simulink model "TST_DrvDem_SetPoint"  (R2016b)
settings: Solver=FixedStepDiscrete  StartTime=0.0  StopTime=simTime  FixedStep=sampleTime  RelTol=1e-3
values from neighbouring files (symbols this model uses):
  testCase = 1    [initTST_DrvDem_SetPoint_001.m]    (also in initTST_DrvDem_SetPoint_002.m = 2; initTST_DrvDem_SetPoint_003.m = 3)
libraries: simulink x13, UnitTest_Lib x9
settings Model: Creator=zhengjinyan  LastModifiedBy=zhengjinyan
settings DebuggingCC: SignalRangeChecking=error

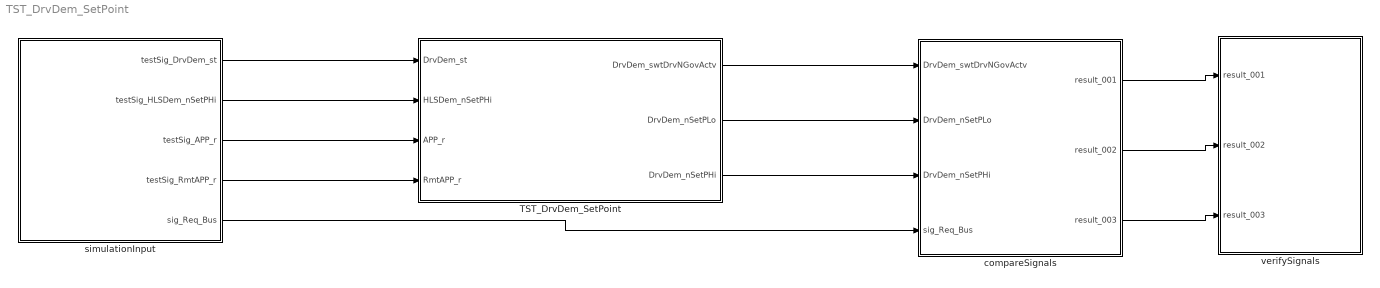
== system TST_DrvDem_SetPoint ==
  TST_DrvDem_SetPoint : Subsystem
  compareSignals : Subsystem
  simulationInput : Subsystem
  verifySignals : Subsystem
  wires:
  simulationInput/1(testSig_DrvDem_st) -> TST_DrvDem_SetPoint/1(DrvDem_st)
  simulationInput/2(testSig_HLSDem_nSetPHi) -> TST_DrvDem_SetPoint/2(HLSDem_nSetPHi)
  simulationInput/3(testSig_APP_r) -> TST_DrvDem_SetPoint/3(APP_r)
  simulationInput/4(testSig_RmtAPP_r) -> TST_DrvDem_SetPoint/4(RmtAPP_r)
  TST_DrvDem_SetPoint/1(DrvDem_swtDrvNGovActv) -> compareSignals/1(DrvDem_swtDrvNGovActv)
  TST_DrvDem_SetPoint/2(DrvDem_nSetPLo) -> compareSignals/2(DrvDem_nSetPLo)
  TST_DrvDem_SetPoint/3(DrvDem_nSetPHi) -> compareSignals/3(DrvDem_nSetPHi)
  simulationInput/5(sig_Req_Bus) -> compareSignals/4(sig_Req_Bus)
  compareSignals/1(result_001) -> verifySignals/1(result_001)
  compareSignals/2(result_002) -> verifySignals/2(result_002)
  compareSignals/3(result_003) -> verifySignals/3(result_003)

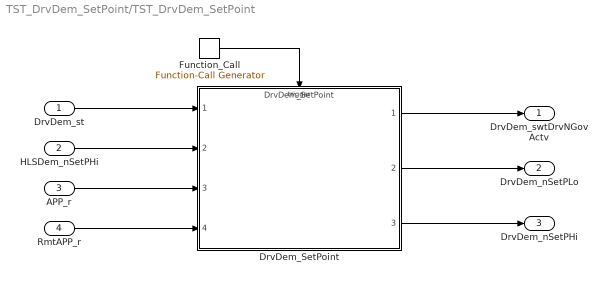
== system TST_DrvDem_SetPoint/TST_DrvDem_SetPoint ==
  DrvDem_st : Inport
  HLSDem_nSetPHi : Inport  Port=2
  APP_r : Inport  Port=3
  RmtAPP_r : Inport  Port=4
  DrvDem_SetPoint : ModelReference  ModelNameDialog=DrvDem_SetPoint  SimulationMode=Normal  ModelReferenceVersion=1.79  TriggerPortName=function  TriggerPortTriggerType=function-call  TriggerPortStatesWhenEnabling=held
  Function_Call : simulink/Ports & Subsystems/Function-Call Generator  sample_time=sampleTime  numberOfIterations=1
  DrvDem_swtDrvNGovActv : Outport
  DrvDem_nSetPLo : Outport  Port=2
  DrvDem_nSetPHi : Outport  Port=3
  wires:
  Function_Call/1 -> DrvDem_SetPoint/Trigger
  DrvDem_st/1 -> DrvDem_SetPoint/1
  HLSDem_nSetPHi/1 -> DrvDem_SetPoint/2
  APP_r/1 -> DrvDem_SetPoint/3
  RmtAPP_r/1 -> DrvDem_SetPoint/4
  DrvDem_SetPoint/1 -> DrvDem_swtDrvNGovActv/1
  DrvDem_SetPoint/2 -> DrvDem_nSetPLo/1
  DrvDem_SetPoint/3 -> DrvDem_nSetPHi/1

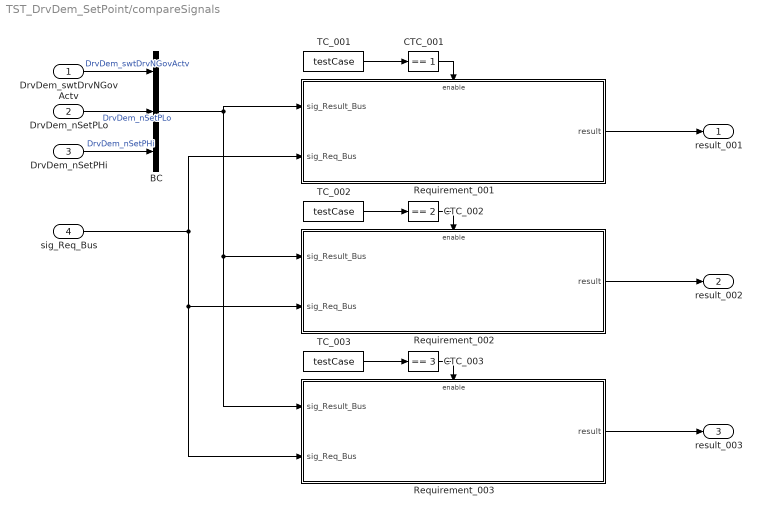
== system TST_DrvDem_SetPoint/compareSignals ==
  DrvDem_swtDrvNGovActv : Inport
  DrvDem_nSetPLo : Inport  Port=2
  DrvDem_nSetPHi : Inport  Port=3
  sig_Req_Bus : Inport  Port=4
  BC : BusCreator  Inputs=3
  CTC_001 : simulink/Logic and Bit Operations/Compare To Constant  relop===  const=1  OutDataTypeStr=boolean
  CTC_002 : simulink/Logic and Bit Operations/Compare To Constant  relop===  const=2  OutDataTypeStr=boolean
  CTC_003 : simulink/Logic and Bit Operations/Compare To Constant  relop===  const=3  OutDataTypeStr=boolean
  Requirement_001 : Subsystem
  Requirement_002 : Subsystem
  Requirement_003 : Subsystem
  TC_001 : Constant  Value=testCase
  TC_002 : Constant  Value=testCase
  TC_003 : Constant  Value=testCase
  result_001 : Outport
  result_002 : Outport  Port=2
  result_003 : Outport  Port=3
  wires:
  DrvDem_swtDrvNGovActv/1 -> BC/1  "DrvDem_swtDrvNGovActv"
  DrvDem_nSetPLo/1 -> BC/2  "DrvDem_nSetPLo"
  DrvDem_nSetPHi/1 -> BC/3  "DrvDem_nSetPHi"
  TC_001/1 -> CTC_001/1
  CTC_001/1 -> Requirement_001/Enable
  sig_Req_Bus/1 -> Requirement_002/2(sig_Req_Bus), Requirement_003/2(sig_Req_Bus), Requirement_001/2(sig_Req_Bus)
  BC/1 -> Requirement_002/1(sig_Result_Bus), Requirement_003/1(sig_Result_Bus), Requirement_001/1(sig_Result_Bus)
  Requirement_001/1(result) -> result_001/1
  TC_002/1 -> CTC_002/1
  CTC_002/1 -> Requirement_002/Enable
  Requirement_002/1(result) -> result_002/1
  TC_003/1 -> CTC_003/1
  CTC_003/1 -> Requirement_003/Enable
  Requirement_003/1(result) -> result_003/1

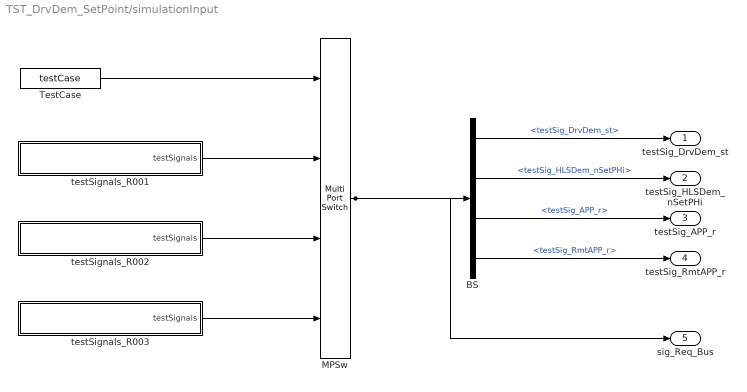
== system TST_DrvDem_SetPoint/simulationInput ==
  BS : BusSelector  OutputSignals=testSig_DrvDem_st,testSig_HLSDem_nSetPHi,testSig_APP_r,testSig_RmtAPP_r
  MPSw : MultiPortSwitch  SaturateOnIntegerOverflow=on  InputSameDT=on
  TestCase : Constant  Value=testCase
  testSignals_R001 : Subsystem
  testSignals_R002 : Subsystem
  testSignals_R003 : Subsystem
  testSig_DrvDem_st : Outport
  testSig_HLSDem_nSetPHi : Outport  Port=2
  testSig_APP_r : Outport  Port=3
  testSig_RmtAPP_r : Outport  Port=4
  sig_Req_Bus : Outport  Port=5
  wires:
  BS/1 -> testSig_DrvDem_st/1  "<testSig_DrvDem_st>"
  BS/2 -> testSig_HLSDem_nSetPHi/1  "<testSig_HLSDem_nSetPHi>"
  BS/3 -> testSig_APP_r/1  "<testSig_APP_r>"
  BS/4 -> testSig_RmtAPP_r/1  "<testSig_RmtAPP_r>"
  MPSw/1 -> BS/1, sig_Req_Bus/1
  TestCase/1 -> MPSw/1
  testSignals_R001/1(testSignals) -> MPSw/2
  testSignals_R002/1(testSignals) -> MPSw/3
  testSignals_R003/1(testSignals) -> MPSw/4

== system TST_DrvDem_SetPoint/verifySignals ==
  result_001 : Inport
  result_002 : Inport  Port=2
  result_003 : Inport  Port=3
  Assertion_001 : Assertion  Enabled=off
  Assertion_002 : Assertion  Enabled=off
  Assertion_003 : Assertion  Enabled=off
  wires:
  result_001/1 -> Assertion_001/1
  result_002/1 -> Assertion_002/1
  result_003/1 -> Assertion_003/1

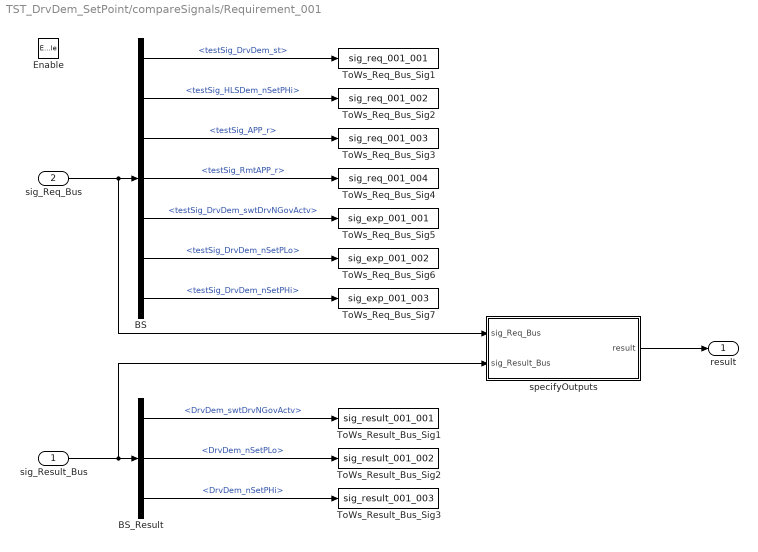
== system TST_DrvDem_SetPoint/compareSignals/Requirement_001 ==
  sig_Result_Bus : Inport
  sig_Req_Bus : Inport  Port=2
  Enable : EnablePort
  BS : BusSelector  OutputSignals=testSig_DrvDem_st,testSig_HLSDem_nSetPHi,testSig_APP_r,testSig_RmtAPP_r,testSig_DrvDem_swtDrvNGovActv,testSig_DrvDem_nSetPLo,testSig_DrvDem_nSetPHi
  BS_Result : BusSelector  OutputSignals=DrvDem_swtDrvNGovActv,DrvDem_nSetPLo,DrvDem_nSetPHi
  ToWs_Req_Bus_Sig1 : ToWorkspace  VariableName=sig_req_001_001  SaveFormat=Structure With Time
  ToWs_Req_Bus_Sig2 : ToWorkspace  VariableName=sig_req_001_002  SaveFormat=Structure With Time
  ToWs_Req_Bus_Sig3 : ToWorkspace  VariableName=sig_req_001_003  SaveFormat=Structure With Time
  ToWs_Req_Bus_Sig4 : ToWorkspace  VariableName=sig_req_001_004  SaveFormat=Structure With Time
  ToWs_Req_Bus_Sig5 : ToWorkspace  VariableName=sig_exp_001_001  SaveFormat=Structure With Time
  ToWs_Req_Bus_Sig6 : ToWorkspace  VariableName=sig_exp_001_002  SaveFormat=Structure With Time
  ToWs_Req_Bus_Sig7 : ToWorkspace  VariableName=sig_exp_001_003  SaveFormat=Structure With Time
  ToWs_Result_Bus_Sig1 : ToWorkspace  VariableName=sig_result_001_001  SaveFormat=Structure With Time
  ToWs_Result_Bus_Sig2 : ToWorkspace  VariableName=sig_result_001_002  SaveFormat=Structure With Time
  ToWs_Result_Bus_Sig3 : ToWorkspace  VariableName=sig_result_001_003  SaveFormat=Structure With Time
  specifyOutputs : Subsystem
  result : Outport
  wires:
  sig_Req_Bus/1 -> BS/1, specifyOutputs/1(sig_Req_Bus)
  BS/1 -> ToWs_Req_Bus_Sig1/1  "<testSig_DrvDem_st>"
  BS/2 -> ToWs_Req_Bus_Sig2/1  "<testSig_HLSDem_nSetPHi>"
  BS/3 -> ToWs_Req_Bus_Sig3/1  "<testSig_APP_r>"
  BS/4 -> ToWs_Req_Bus_Sig4/1  "<testSig_RmtAPP_r>"
  BS/5 -> ToWs_Req_Bus_Sig5/1  "<testSig_DrvDem_swtDrvNGovActv>"
  BS/6 -> ToWs_Req_Bus_Sig6/1  "<testSig_DrvDem_nSetPLo>"
  BS/7 -> ToWs_Req_Bus_Sig7/1  "<testSig_DrvDem_nSetPHi>"
  sig_Result_Bus/1 -> BS_Result/1, specifyOutputs/2(sig_Result_Bus)
  BS_Result/1 -> ToWs_Result_Bus_Sig1/1  "<DrvDem_swtDrvNGovActv>"
  BS_Result/2 -> ToWs_Result_Bus_Sig2/1  "<DrvDem_nSetPLo>"
  BS_Result/3 -> ToWs_Result_Bus_Sig3/1  "<DrvDem_nSetPHi>"
  specifyOutputs/1(result) -> result/1

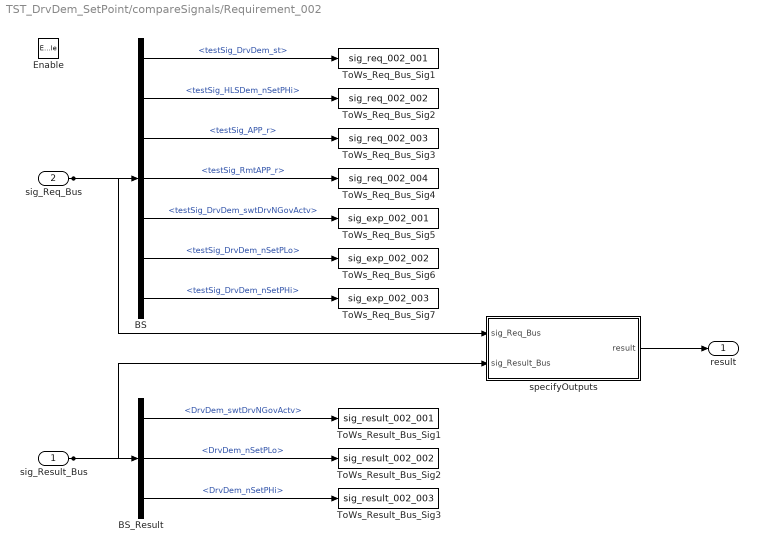
== system TST_DrvDem_SetPoint/compareSignals/Requirement_002 ==
  sig_Result_Bus : Inport
  sig_Req_Bus : Inport  Port=2
  Enable : EnablePort
  BS : BusSelector  OutputSignals=testSig_DrvDem_st,testSig_HLSDem_nSetPHi,testSig_APP_r,testSig_RmtAPP_r,testSig_DrvDem_swtDrvNGovActv,testSig_DrvDem_nSetPLo,testSig_DrvDem_nSetPHi
  BS_Result : BusSelector  OutputSignals=DrvDem_swtDrvNGovActv,DrvDem_nSetPLo,DrvDem_nSetPHi
  ToWs_Req_Bus_Sig1 : ToWorkspace  VariableName=sig_req_002_001  SaveFormat=Structure With Time
  ToWs_Req_Bus_Sig2 : ToWorkspace  VariableName=sig_req_002_002  SaveFormat=Structure With Time
  ToWs_Req_Bus_Sig3 : ToWorkspace  VariableName=sig_req_002_003  SaveFormat=Structure With Time
  ToWs_Req_Bus_Sig4 : ToWorkspace  VariableName=sig_req_002_004  SaveFormat=Structure With Time
  ToWs_Req_Bus_Sig5 : ToWorkspace  VariableName=sig_exp_002_001  SaveFormat=Structure With Time
  ToWs_Req_Bus_Sig6 : ToWorkspace  VariableName=sig_exp_002_002  SaveFormat=Structure With Time
  ToWs_Req_Bus_Sig7 : ToWorkspace  VariableName=sig_exp_002_003  SaveFormat=Structure With Time
  ToWs_Result_Bus_Sig1 : ToWorkspace  VariableName=sig_result_002_001  SaveFormat=Structure With Time
  ToWs_Result_Bus_Sig2 : ToWorkspace  VariableName=sig_result_002_002  SaveFormat=Structure With Time
  ToWs_Result_Bus_Sig3 : ToWorkspace  VariableName=sig_result_002_003  SaveFormat=Structure With Time
  specifyOutputs : Subsystem
  result : Outport
  wires:
  sig_Req_Bus/1 -> BS/1, specifyOutputs/1(sig_Req_Bus)
  BS/1 -> ToWs_Req_Bus_Sig1/1  "<testSig_DrvDem_st>"
  BS/2 -> ToWs_Req_Bus_Sig2/1  "<testSig_HLSDem_nSetPHi>"
  BS/3 -> ToWs_Req_Bus_Sig3/1  "<testSig_APP_r>"
  BS/4 -> ToWs_Req_Bus_Sig4/1  "<testSig_RmtAPP_r>"
  BS/5 -> ToWs_Req_Bus_Sig5/1  "<testSig_DrvDem_swtDrvNGovActv>"
  BS/6 -> ToWs_Req_Bus_Sig6/1  "<testSig_DrvDem_nSetPLo>"
  BS/7 -> ToWs_Req_Bus_Sig7/1  "<testSig_DrvDem_nSetPHi>"
  sig_Result_Bus/1 -> BS_Result/1, specifyOutputs/2(sig_Result_Bus)
  BS_Result/1 -> ToWs_Result_Bus_Sig1/1  "<DrvDem_swtDrvNGovActv>"
  BS_Result/2 -> ToWs_Result_Bus_Sig2/1  "<DrvDem_nSetPLo>"
  BS_Result/3 -> ToWs_Result_Bus_Sig3/1  "<DrvDem_nSetPHi>"
  specifyOutputs/1(result) -> result/1

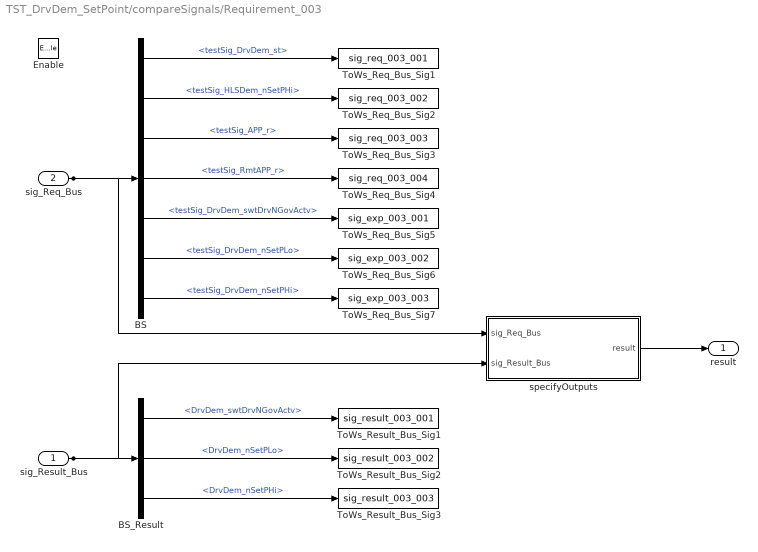
== system TST_DrvDem_SetPoint/compareSignals/Requirement_003 ==
  sig_Result_Bus : Inport
  sig_Req_Bus : Inport  Port=2
  Enable : EnablePort
  BS : BusSelector  OutputSignals=testSig_DrvDem_st,testSig_HLSDem_nSetPHi,testSig_APP_r,testSig_RmtAPP_r,testSig_DrvDem_swtDrvNGovActv,testSig_DrvDem_nSetPLo,testSig_DrvDem_nSetPHi
  BS_Result : BusSelector  OutputSignals=DrvDem_swtDrvNGovActv,DrvDem_nSetPLo,DrvDem_nSetPHi
  ToWs_Req_Bus_Sig1 : ToWorkspace  VariableName=sig_req_003_001  SaveFormat=Structure With Time
  ToWs_Req_Bus_Sig2 : ToWorkspace  VariableName=sig_req_003_002  SaveFormat=Structure With Time
  ToWs_Req_Bus_Sig3 : ToWorkspace  VariableName=sig_req_003_003  SaveFormat=Structure With Time
  ToWs_Req_Bus_Sig4 : ToWorkspace  VariableName=sig_req_003_004  SaveFormat=Structure With Time
  ToWs_Req_Bus_Sig5 : ToWorkspace  VariableName=sig_exp_003_001  SaveFormat=Structure With Time
  ToWs_Req_Bus_Sig6 : ToWorkspace  VariableName=sig_exp_003_002  SaveFormat=Structure With Time
  ToWs_Req_Bus_Sig7 : ToWorkspace  VariableName=sig_exp_003_003  SaveFormat=Structure With Time
  ToWs_Result_Bus_Sig1 : ToWorkspace  VariableName=sig_result_003_001  SaveFormat=Structure With Time
  ToWs_Result_Bus_Sig2 : ToWorkspace  VariableName=sig_result_003_002  SaveFormat=Structure With Time
  ToWs_Result_Bus_Sig3 : ToWorkspace  VariableName=sig_result_003_003  SaveFormat=Structure With Time
  specifyOutputs : Subsystem
  result : Outport
  wires:
  sig_Req_Bus/1 -> BS/1, specifyOutputs/1(sig_Req_Bus)
  BS/1 -> ToWs_Req_Bus_Sig1/1  "<testSig_DrvDem_st>"
  BS/2 -> ToWs_Req_Bus_Sig2/1  "<testSig_HLSDem_nSetPHi>"
  BS/3 -> ToWs_Req_Bus_Sig3/1  "<testSig_APP_r>"
  BS/4 -> ToWs_Req_Bus_Sig4/1  "<testSig_RmtAPP_r>"
  BS/5 -> ToWs_Req_Bus_Sig5/1  "<testSig_DrvDem_swtDrvNGovActv>"
  BS/6 -> ToWs_Req_Bus_Sig6/1  "<testSig_DrvDem_nSetPLo>"
  BS/7 -> ToWs_Req_Bus_Sig7/1  "<testSig_DrvDem_nSetPHi>"
  sig_Result_Bus/1 -> BS_Result/1, specifyOutputs/2(sig_Result_Bus)
  BS_Result/1 -> ToWs_Result_Bus_Sig1/1  "<DrvDem_swtDrvNGovActv>"
  BS_Result/2 -> ToWs_Result_Bus_Sig2/1  "<DrvDem_nSetPLo>"
  BS_Result/3 -> ToWs_Result_Bus_Sig3/1  "<DrvDem_nSetPHi>"
  specifyOutputs/1(result) -> result/1

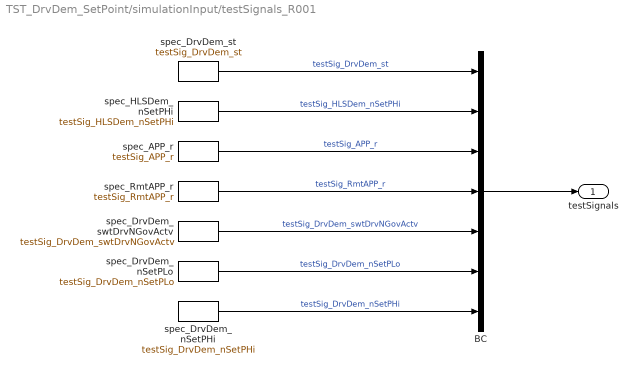
== system TST_DrvDem_SetPoint/simulationInput/testSignals_R001 ==
  BC : BusCreator  Inputs=7
  spec_APP_r : FromWorkspace  VariableName=testSig_APP_r  Interpolate=off  OutputAfterFinalValue=Holding final value
  spec_DrvDem_nSetPHi : FromWorkspace  VariableName=testSig_DrvDem_nSetPHi  Interpolate=off  OutputAfterFinalValue=Holding final value
  spec_DrvDem_nSetPLo : FromWorkspace  VariableName=testSig_DrvDem_nSetPLo  Interpolate=off  OutputAfterFinalValue=Holding final value
  spec_DrvDem_st : FromWorkspace  VariableName=testSig_DrvDem_st  Interpolate=off  OutputAfterFinalValue=Holding final value
  spec_DrvDem_swtDrvNGovActv : FromWorkspace  VariableName=testSig_DrvDem_swtDrvNGovActv  Interpolate=off  OutputAfterFinalValue=Holding final value
  spec_HLSDem_nSetPHi : FromWorkspace  VariableName=testSig_HLSDem_nSetPHi  Interpolate=off  OutputAfterFinalValue=Holding final value
  spec_RmtAPP_r : FromWorkspace  VariableName=testSig_RmtAPP_r  Interpolate=off  OutputAfterFinalValue=Holding final value
  testSignals : Outport
  wires:
  BC/1 -> testSignals/1
  spec_DrvDem_st/1 -> BC/1  "testSig_DrvDem_st"
  spec_HLSDem_nSetPHi/1 -> BC/2  "testSig_HLSDem_nSetPHi"
  spec_APP_r/1 -> BC/3  "testSig_APP_r"
  spec_RmtAPP_r/1 -> BC/4  "testSig_RmtAPP_r"
  spec_DrvDem_swtDrvNGovActv/1 -> BC/5  "testSig_DrvDem_swtDrvNGovActv"
  spec_DrvDem_nSetPLo/1 -> BC/6  "testSig_DrvDem_nSetPLo"
  spec_DrvDem_nSetPHi/1 -> BC/7  "testSig_DrvDem_nSetPHi"

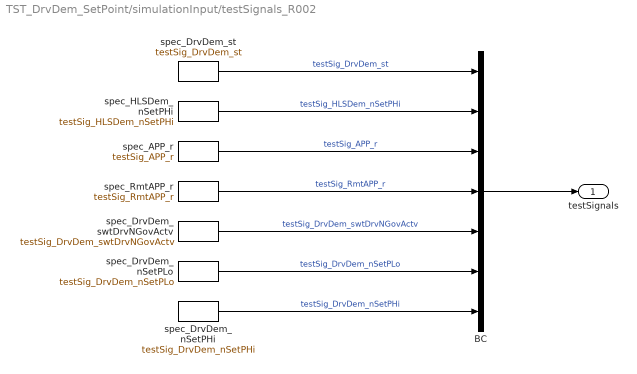
== system TST_DrvDem_SetPoint/simulationInput/testSignals_R002 ==
  BC : BusCreator  Inputs=7
  spec_APP_r : FromWorkspace  VariableName=testSig_APP_r  Interpolate=off  OutputAfterFinalValue=Holding final value
  spec_DrvDem_nSetPHi : FromWorkspace  VariableName=testSig_DrvDem_nSetPHi  Interpolate=off  OutputAfterFinalValue=Holding final value
  spec_DrvDem_nSetPLo : FromWorkspace  VariableName=testSig_DrvDem_nSetPLo  Interpolate=off  OutputAfterFinalValue=Holding final value
  spec_DrvDem_st : FromWorkspace  VariableName=testSig_DrvDem_st  Interpolate=off  OutputAfterFinalValue=Holding final value
  spec_DrvDem_swtDrvNGovActv : FromWorkspace  VariableName=testSig_DrvDem_swtDrvNGovActv  Interpolate=off  OutputAfterFinalValue=Holding final value
  spec_HLSDem_nSetPHi : FromWorkspace  VariableName=testSig_HLSDem_nSetPHi  Interpolate=off  OutputAfterFinalValue=Holding final value
  spec_RmtAPP_r : FromWorkspace  VariableName=testSig_RmtAPP_r  Interpolate=off  OutputAfterFinalValue=Holding final value
  testSignals : Outport
  wires:
  BC/1 -> testSignals/1
  spec_DrvDem_st/1 -> BC/1  "testSig_DrvDem_st"
  spec_HLSDem_nSetPHi/1 -> BC/2  "testSig_HLSDem_nSetPHi"
  spec_APP_r/1 -> BC/3  "testSig_APP_r"
  spec_RmtAPP_r/1 -> BC/4  "testSig_RmtAPP_r"
  spec_DrvDem_swtDrvNGovActv/1 -> BC/5  "testSig_DrvDem_swtDrvNGovActv"
  spec_DrvDem_nSetPLo/1 -> BC/6  "testSig_DrvDem_nSetPLo"
  spec_DrvDem_nSetPHi/1 -> BC/7  "testSig_DrvDem_nSetPHi"

== system TST_DrvDem_SetPoint/simulationInput/testSignals_R003 ==
  BC : BusCreator  Inputs=7
  spec_APP_r : FromWorkspace  VariableName=testSig_APP_r  Interpolate=off  OutputAfterFinalValue=Holding final value
  spec_DrvDem_nSetPHi : FromWorkspace  VariableName=testSig_DrvDem_nSetPHi  Interpolate=off  OutputAfterFinalValue=Holding final value
  spec_DrvDem_nSetPLo : FromWorkspace  VariableName=testSig_DrvDem_nSetPLo  Interpolate=off  OutputAfterFinalValue=Holding final value
  spec_DrvDem_st : FromWorkspace  VariableName=testSig_DrvDem_st  Interpolate=off  OutputAfterFinalValue=Holding final value
  spec_DrvDem_swtDrvNGovActv : FromWorkspace  VariableName=testSig_DrvDem_swtDrvNGovActv  Interpolate=off  OutputAfterFinalValue=Holding final value
  spec_HLSDem_nSetPHi : FromWorkspace  VariableName=testSig_HLSDem_nSetPHi  Interpolate=off  OutputAfterFinalValue=Holding final value
  spec_RmtAPP_r : FromWorkspace  VariableName=testSig_RmtAPP_r  Interpolate=off  OutputAfterFinalValue=Holding final value
  testSignals : Outport
  wires:
  BC/1 -> testSignals/1
  spec_DrvDem_st/1 -> BC/1  "testSig_DrvDem_st"
  spec_HLSDem_nSetPHi/1 -> BC/2  "testSig_HLSDem_nSetPHi"
  spec_APP_r/1 -> BC/3  "testSig_APP_r"
  spec_RmtAPP_r/1 -> BC/4  "testSig_RmtAPP_r"
  spec_DrvDem_swtDrvNGovActv/1 -> BC/5  "testSig_DrvDem_swtDrvNGovActv"
  spec_DrvDem_nSetPLo/1 -> BC/6  "testSig_DrvDem_nSetPLo"
  spec_DrvDem_nSetPHi/1 -> BC/7  "testSig_DrvDem_nSetPHi"

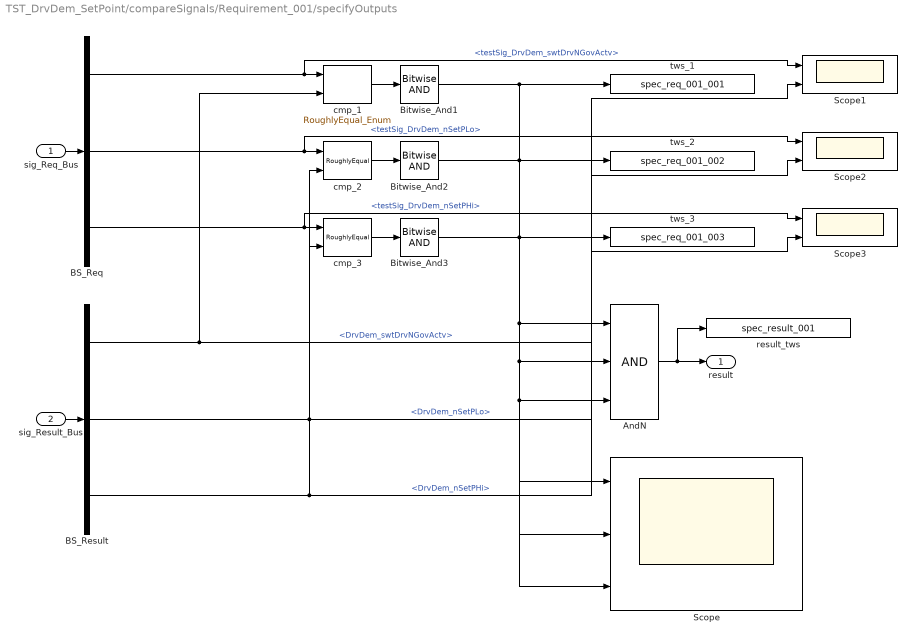
== system TST_DrvDem_SetPoint/compareSignals/Requirement_001/specifyOutputs ==
  sig_Req_Bus : Inport
  sig_Result_Bus : Inport  Port=2
  AndN : Logic  Inputs=3
  BS_Req : BusSelector  OutputSignals=testSig_DrvDem_swtDrvNGovActv,testSig_DrvDem_nSetPLo,testSig_DrvDem_nSetPHi
  BS_Result : BusSelector  OutputSignals=DrvDem_swtDrvNGovActv,DrvDem_nSetPLo,DrvDem_nSetPHi
  Bitwise_And1 : simulink/Logic and Bit Operations/Bitwise Operator  logicop=AND  UseBitMask=off  BitMask=bin2dec('11011001')  BitMaskRealWorld=Stored Integer
  Bitwise_And2 : simulink/Logic and Bit Operations/Bitwise Operator  logicop=AND  UseBitMask=off  BitMask=bin2dec('11011001')  BitMaskRealWorld=Stored Integer
  Bitwise_And3 : simulink/Logic and Bit Operations/Bitwise Operator  logicop=AND  UseBitMask=off  BitMask=bin2dec('11011001')  BitMaskRealWorld=Stored Integer
  Scope : Scope  NumInputPorts=3
  Scope1 : Scope  NumInputPorts=2
  Scope2 : Scope  NumInputPorts=2
  Scope3 : Scope  NumInputPorts=2
  cmp_1 : UnitTest_Lib/RoughlyEqual_Enum  slope=0.1
  cmp_2 : UnitTest_Lib/RoughlyEqual  slope=2
  cmp_3 : UnitTest_Lib/RoughlyEqual  slope=0.1
  result_tws : ToWorkspace  VariableName=spec_result_001
  tws_1 : ToWorkspace  VariableName=spec_req_001_001
  tws_2 : ToWorkspace  VariableName=spec_req_001_002
  tws_3 : ToWorkspace  VariableName=spec_req_001_003
  result : Outport
  wires:
  sig_Req_Bus/1 -> BS_Req/1
  sig_Result_Bus/1 -> BS_Result/1
  AndN/1 -> result/1, result_tws/1
  BS_Req/1 -> cmp_1/1, Scope1/1  "<testSig_DrvDem_swtDrvNGovActv>"
  BS_Result/1 -> cmp_1/2, Scope1/2  "<DrvDem_swtDrvNGovActv>"
  cmp_1/1 -> Bitwise_And1/1
  Bitwise_And1/1 -> AndN/1, Scope/1, tws_1/1
  BS_Req/2 -> cmp_2/1, Scope2/1  "<testSig_DrvDem_nSetPLo>"
  BS_Result/2 -> cmp_2/2, Scope2/2  "<DrvDem_nSetPLo>"
  cmp_2/1 -> Bitwise_And2/1
  Bitwise_And2/1 -> AndN/2, Scope/2, tws_2/1
  BS_Req/3 -> cmp_3/1, Scope3/1  "<testSig_DrvDem_nSetPHi>"
  BS_Result/3 -> cmp_3/2, Scope3/2  "<DrvDem_nSetPHi>"
  cmp_3/1 -> Bitwise_And3/1
  Bitwise_And3/1 -> AndN/3, Scope/3, tws_3/1

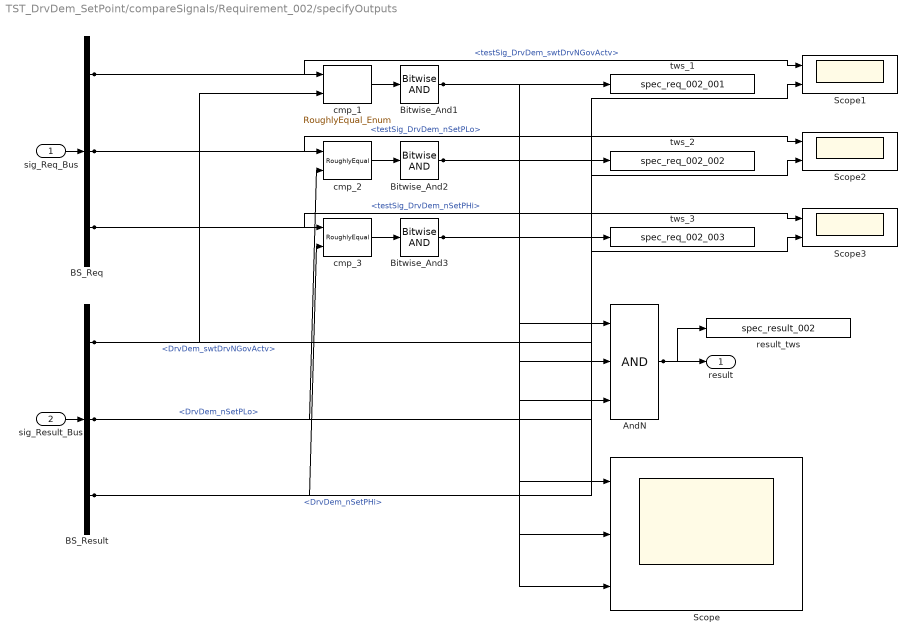
== system TST_DrvDem_SetPoint/compareSignals/Requirement_002/specifyOutputs ==
  sig_Req_Bus : Inport
  sig_Result_Bus : Inport  Port=2
  AndN : Logic  Inputs=3
  BS_Req : BusSelector  OutputSignals=testSig_DrvDem_swtDrvNGovActv,testSig_DrvDem_nSetPLo,testSig_DrvDem_nSetPHi
  BS_Result : BusSelector  OutputSignals=DrvDem_swtDrvNGovActv,DrvDem_nSetPLo,DrvDem_nSetPHi
  Bitwise_And1 : simulink/Logic and Bit Operations/Bitwise Operator  logicop=AND  UseBitMask=off  BitMask=bin2dec('11011001')  BitMaskRealWorld=Stored Integer
  Bitwise_And2 : simulink/Logic and Bit Operations/Bitwise Operator  logicop=AND  UseBitMask=off  BitMask=bin2dec('11011001')  BitMaskRealWorld=Stored Integer
  Bitwise_And3 : simulink/Logic and Bit Operations/Bitwise Operator  logicop=AND  UseBitMask=off  BitMask=bin2dec('11011001')  BitMaskRealWorld=Stored Integer
  Scope : Scope  NumInputPorts=3
  Scope1 : Scope  NumInputPorts=2
  Scope2 : Scope  NumInputPorts=2
  Scope3 : Scope  NumInputPorts=2
  cmp_1 : UnitTest_Lib/RoughlyEqual_Enum  slope=0.1
  cmp_2 : UnitTest_Lib/RoughlyEqual  slope=0.1
  cmp_3 : UnitTest_Lib/RoughlyEqual  slope=0.1
  result_tws : ToWorkspace  VariableName=spec_result_002
  tws_1 : ToWorkspace  VariableName=spec_req_002_001
  tws_2 : ToWorkspace  VariableName=spec_req_002_002
  tws_3 : ToWorkspace  VariableName=spec_req_002_003
  result : Outport
  wires:
  sig_Req_Bus/1 -> BS_Req/1
  sig_Result_Bus/1 -> BS_Result/1
  AndN/1 -> result/1, result_tws/1
  BS_Req/1 -> cmp_1/1, Scope1/1  "<testSig_DrvDem_swtDrvNGovActv>"
  BS_Result/1 -> cmp_1/2, Scope1/2  "<DrvDem_swtDrvNGovActv>"
  cmp_1/1 -> Bitwise_And1/1
  Bitwise_And1/1 -> tws_1/1, AndN/1, Scope/1
  BS_Req/2 -> cmp_2/1, Scope2/1  "<testSig_DrvDem_nSetPLo>"
  BS_Result/2 -> cmp_2/2, Scope2/2  "<DrvDem_nSetPLo>"
  cmp_2/1 -> Bitwise_And2/1
  Bitwise_And2/1 -> tws_2/1, AndN/2, Scope/2
  BS_Req/3 -> cmp_3/1, Scope3/1  "<testSig_DrvDem_nSetPHi>"
  BS_Result/3 -> cmp_3/2, Scope3/2  "<DrvDem_nSetPHi>"
  cmp_3/1 -> Bitwise_And3/1
  Bitwise_And3/1 -> tws_3/1, AndN/3, Scope/3

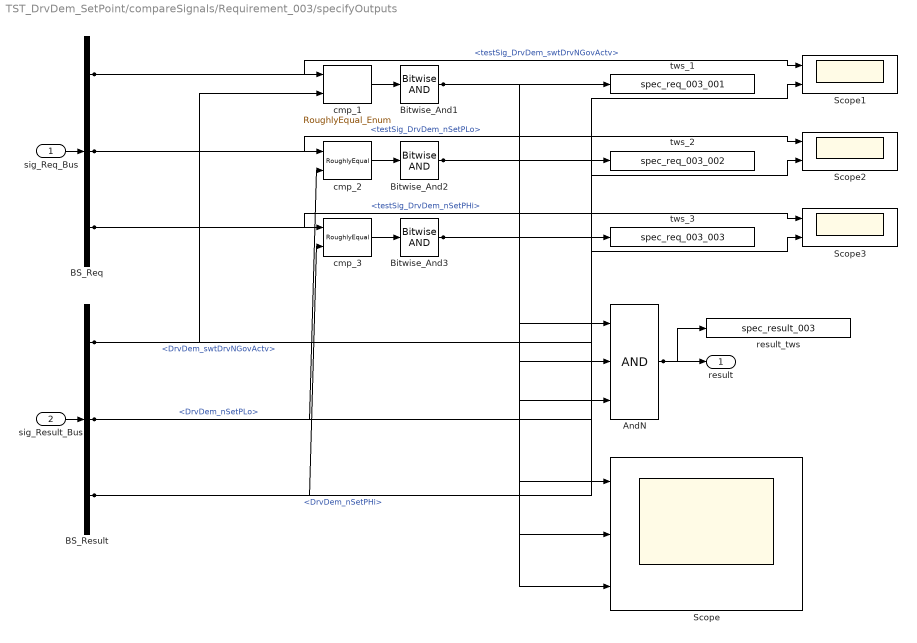
== system TST_DrvDem_SetPoint/compareSignals/Requirement_003/specifyOutputs ==
  sig_Req_Bus : Inport
  sig_Result_Bus : Inport  Port=2
  AndN : Logic  Inputs=3
  BS_Req : BusSelector  OutputSignals=testSig_DrvDem_swtDrvNGovActv,testSig_DrvDem_nSetPLo,testSig_DrvDem_nSetPHi
  BS_Result : BusSelector  OutputSignals=DrvDem_swtDrvNGovActv,DrvDem_nSetPLo,DrvDem_nSetPHi
  Bitwise_And1 : simulink/Logic and Bit Operations/Bitwise Operator  logicop=AND  UseBitMask=off  BitMask=bin2dec('11011001')  BitMaskRealWorld=Stored Integer
  Bitwise_And2 : simulink/Logic and Bit Operations/Bitwise Operator  logicop=AND  UseBitMask=off  BitMask=bin2dec('11011001')  BitMaskRealWorld=Stored Integer
  Bitwise_And3 : simulink/Logic and Bit Operations/Bitwise Operator  logicop=AND  UseBitMask=off  BitMask=bin2dec('11011001')  BitMaskRealWorld=Stored Integer
  Scope : Scope  NumInputPorts=3
  Scope1 : Scope  NumInputPorts=2
  Scope2 : Scope  NumInputPorts=2
  Scope3 : Scope  NumInputPorts=2
  cmp_1 : UnitTest_Lib/RoughlyEqual_Enum  slope=0.1
  cmp_2 : UnitTest_Lib/RoughlyEqual  slope=0.1
  cmp_3 : UnitTest_Lib/RoughlyEqual  slope=0.1
  result_tws : ToWorkspace  VariableName=spec_result_003
  tws_1 : ToWorkspace  VariableName=spec_req_003_001
  tws_2 : ToWorkspace  VariableName=spec_req_003_002
  tws_3 : ToWorkspace  VariableName=spec_req_003_003
  result : Outport
  wires:
  sig_Req_Bus/1 -> BS_Req/1
  sig_Result_Bus/1 -> BS_Result/1
  AndN/1 -> result/1, result_tws/1
  BS_Req/1 -> cmp_1/1, Scope1/1  "<testSig_DrvDem_swtDrvNGovActv>"
  BS_Result/1 -> cmp_1/2, Scope1/2  "<DrvDem_swtDrvNGovActv>"
  cmp_1/1 -> Bitwise_And1/1
  Bitwise_And1/1 -> tws_1/1, AndN/1, Scope/1
  BS_Req/2 -> cmp_2/1, Scope2/1  "<testSig_DrvDem_nSetPLo>"
  BS_Result/2 -> cmp_2/2, Scope2/2  "<DrvDem_nSetPLo>"
  cmp_2/1 -> Bitwise_And2/1
  Bitwise_And2/1 -> tws_2/1, AndN/2, Scope/2
  BS_Req/3 -> cmp_3/1, Scope3/1  "<testSig_DrvDem_nSetPHi>"
  BS_Result/3 -> cmp_3/2, Scope3/2  "<DrvDem_nSetPHi>"
  cmp_3/1 -> Bitwise_And3/1
  Bitwise_And3/1 -> tws_3/1, AndN/3, Scope/3
